simulink model "Simulate_v2"  (R2024b)
settings: Solver=VariableStepAuto  StartTime=0.0  StopTime=Tf  FixedStep=Ti  MaxStep=Ti  RelTol=1e-6
undefined symbols (not defined in the file): CCMPC, CEMPC, DiscIntNeverNeededParam, dspblkCoreblockFVToolHelper, FOC, gcbh, IM, LPF, M2C, plecs, PLL, RFT, TEB, Ti, Ts
libraries: slpidlib x4, dspstat3 x1, embmathops x1, spsabctodq0Lib x1, spsdq0toabcLib x1
settings Model: Creator=Pablo  LastModifiedBy=Pablo

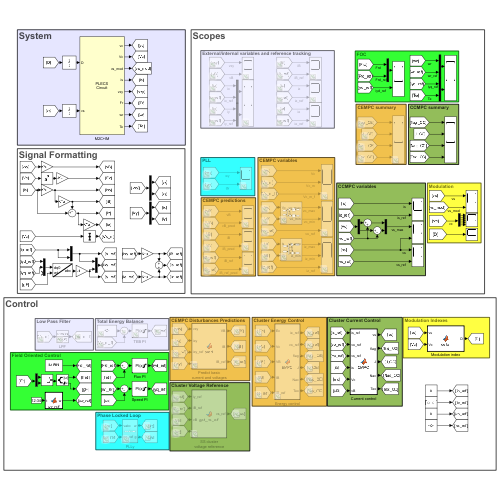
[thumbnail: Simulink's stored preview of the top-level diagram]
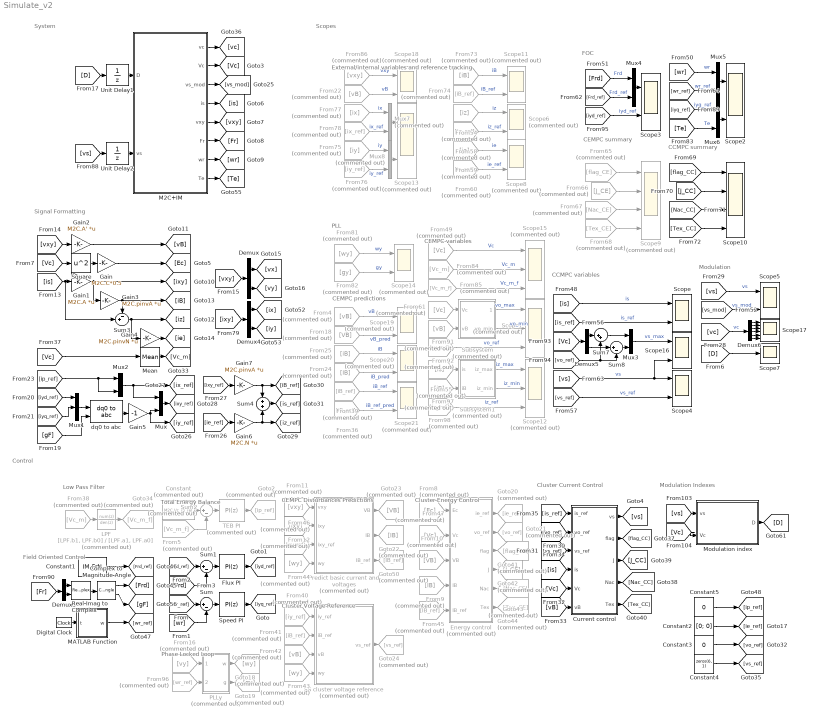
== system Simulate_v2 ==
  note: System
  note: Control
  note: Scopes
  note: External/internal variables and reference tracking
  note: CCMPC variables
  note: PLL
  note: CEMPC variables
  note: CEMPC predictions
  note: Modulation
  note: FOC
  note: CEMPC summary
  note: Cluster Current Control
  note: Cluster Voltage Reference
  note: Cluster Energy Control
  note: Signal Formatting
  note: CEMPC Disturbances Predictions
  note: Field Oriented Control
  note: Total Energy Balance
  note: Low Pass Filter
  note: Phase Locked Loop
  note: CCMPC summary
  note: Modulation Indexes
  Complex to Magnitude-Angle : ComplexToMagnitudeAngle
  Constant : Constant  Commented=on  Value=M2C.Vc_m_ref  SampleTime=Ts
  Constant1 : Constant  Value=IM.FrN  SampleTime=Ts
  Constant2 : Constant  Value=[0; 0]  SampleTime=Ts
  Constant3 : Constant  Value=0  SampleTime=Ts
  Constant4 : Constant  Value=zeros(6, 1)  SampleTime=Ts
  Constant5 : Constant  Value=0  SampleTime=Ts
  Current control : MATLAB Function  TreatAsAtomicUnit=on  SystemSampleTime=CCMPC.Ts
  Demux : Demux  Outputs=[2; 3]
  Demux3 : Demux  Outputs=2
  Demux4 : Demux  Outputs=[2; 3]
  Demux5 : Demux  Outputs=[3; 3]
  Demux6 : Demux  Outputs=M2C.m
  Digital Clock : DigitalClock  SampleTime=Ts
  Energy control : MATLAB Function  Commented=on  TreatAsAtomicUnit=on  SystemSampleTime=CEMPC.Ts
  Flux PI : slpidlib/PID Controller  Controller=PI  Form=Parallel  TimeDomain=Discrete-time  UseExternalTs=off  SampleTime=FOC.Ts  IntegratorMethod=Forward Euler  FilterMethod=Forward Euler  ControllerParametersSource=internal  P=FOC.kp_F  I=FOC.ki_F  UseKiTs=off  D=0  UseExternalDerivativeSource=off  N=100  UseFilter=on  TunerSelectOption=Transfer Function Based (PID Tuner App)  InitialConditionSource=internal  InitialConditionForIntegrator=0  InitialConditionForFilter=0  DifferentiatorICPrevScaledInput=0  ExternalReset=none  TrackingMode=off  Kt=1  LimitOutput=on  SatLimitsSource=internal  UpperSaturationLimit=FOC.u_max  LowerSaturationLimit=FOC.u_min  LinearizeAsGain=on  AntiWindupMode=back-calculation  Kb=FOC.kp_F  LimitIntegrator=off  UpperIntegratorSaturationLimit=inf  LowerIntegratorSaturationLimit=-inf  POutMin=[]  POutMax=[]  IOutMin=[]  IOutMax=[]  DOutMin=[]  DOutMax=[]  NOutMin=[]  NOutMax=[]  SumOutMin=[]  SumOutMax=[]  SaturationOutMin=[]  SaturationOutMax=[]  PParamMin=[]  PParamMax=[]  IParamMin=[]  IParamMax=[]  DParamMin=[]  DParamMax=[]  NParamMin=[]  NParamMax=[]  KbParamMin=[]  KbParamMax=[]  KtParamMin=[]  KtParamMax=[]  KbOutMin=[]  KbOutMax=[]  KtOutMin=[]  KtOutMax=[]  IntegratorOutMin=[]  IntegratorOutMax=[]  FilterOutMin=[]  FilterOutMax=[]  SumI1OutMin=[]  SumI1OutMax=[]  SumI2OutMin=[]  SumI2OutMax=[]  SumI3OutMin=[]  SumI3OutMax=[]  SumI4OutMin=[]  SumI4OutMax=[]  SumDOutMin=[]  SumDOutMax=[]  DifferentiatorOutMin=[]  DifferentiatorOutMax=[]  FilterDiffOutCoefMin=[]  FilterDiffOutCoefMax=[]  ReciprocalOutMin=[]  ReciprocalOutMax=[]  SumDenOutMin=[]  SumDenOutMax=[]  SumNumOutMin=[]  SumNumOutMax=[]  DivideOutMin=[]  DivideOutMax=[]  UdiffTsProdOutMin=[]  UdiffTsProdOutMax=[]  NTsProdOutMin=[]  NTsProdOutMax=[]  UintegralTsProdOutMin=[]  UintegralTsProdOutMax=[]  UngainTsProdOutMin=[]  UngainTsProdOutMax=[]  ClampingZeroOutDataTypeStr=Inherit: Inherit via back propagation  ClampingZeroOutMin=[]  ClampingZeroOutMax=[]  FilterDenConstantOutDataTypeStr=Inherit: Inherit via back propagation  FilterDenConstantOutMin=[]  FilterDenConstantOutMax=[]  PCopyOutDataTypeStr=Inherit: Inherit via back propagation  PCopyOutMin=[]  PCopyOutMax=[]  NCopyOutDataTypeStr=Inherit: Inherit via back propagation  NCopyOutMin=[]  NCopyOutMax=[]  IntegratorContinuousStateAttributes=''  IntegratorStateMustResolveToSignalObject=off  IntegratorRTWStateStorageClass=Auto  FilterContinuousStateAttributes=''  FilterStateMustResolveToSignalObject=off  FilterRTWStateStorageClass=Auto  ParallelPVariant=InternalParameters  IdealPVariant=Disabled  IVariant=InternalParameters  DVariant=Disabled  IntegratorVariant=Discrete  SatVariant=Enabled  AWVariant=BackCalculation  PCopyVariant=Disabled  TRVariant=Disabled  FdbkBlocksVariant=Forward  IdealPFdbkVariant=Disabled  SatFdbkVariant=Disabled  DerivativeFilterVariant=Disabled  NVariant=Disabled  NCopyVariant=Disabled_SignalSpec  FilterICVariant=Disabled  IntegratorICVariant=InternalICs  ExternalResetVariant=Disabled  TRSumVariant=Passthrough  SumFdbkVariant=Disabled  SumVariant=Sum_PI  TsampFilterVariant=InternalTs  TsampNgainVariant=Passthrough  TsampIntegralVariant=Disabled_SignalSpec  ExternalSaturationOutDataTypeStr=Inherit: Same as second input  DerivativeSourceVariant=Disabled  PreIntVariant=InternalPreInt
  From10 : From  Commented=on  GotoTag=VB
  From11 : From  Commented=on  GotoTag=vxy
  From12 : From  Commented=on  GotoTag=ixy
  From16 : From  Commented=on  GotoTag=vy
  From18 : From  Commented=on  GotoTag=VB
  From{4,22,42,91} (4 alike) : From  Commented=on  GotoTag=vB
  From24 : From  Commented=on  GotoTag=IB
  From25 : From  Commented=on  GotoTag=iB
  From36 : From  Commented=on  GotoTag=IB_ref
  From38 : From  Commented=on  GotoTag=Vc_m
  From39 : From  Commented=on  GotoTag=iB_ref
  From40 : From  Commented=on  GotoTag=iy_ref
  From41 : From  Commented=on  GotoTag=iB_ref
  From43 : From  Commented=on  GotoTag=wy
  From44 : From  Commented=on  GotoTag=wy
  From45 : From  Commented=on  GotoTag=IB_ref
  From46 : From  Commented=on  GotoTag=ixy_ref
  From47 : From  Commented=on  GotoTag=Vc
  From49 : From  Commented=on  GotoTag=Vc
  From5 : From  Commented=on  GotoTag=Vc_m_f
  From54 : From  Commented=on  GotoTag=iz
  From55 : From  Commented=on  GotoTag=is
  From58 : From  Commented=on  GotoTag=iz_ref
  From59 : From  Commented=on  GotoTag=ie
  From60 : From  Commented=on  GotoTag=ie_ref
  From61 : From  Commented=on  GotoTag=Vc
  From65 : From  Commented=on  GotoTag=flag_CE
  From66 : From  Commented=on  GotoTag=J_CE
  From67 : From  Commented=on  GotoTag=Nac_CE
  From68 : From  Commented=on  GotoTag=Tex_CE
  From73 : From  Commented=on  GotoTag=iB
  From74 : From  Commented=on  GotoTag=iB_ref
  From75 : From  Commented=on  GotoTag=iy
  From76 : From  Commented=on  GotoTag=iy_ref
  From77 : From  Commented=on  GotoTag=ix
  From78 : From  Commented=on  GotoTag=ix_ref
  From8 : From  Commented=on  GotoTag=Ec
  From81 : From  Commented=on  GotoTag=wy
  From82 : From  Commented=on  GotoTag=gy
  From84 : From  Commented=on  GotoTag=Vc_m
  From85 : From  Commented=on  GotoTag=Vc_m_f
  From86 : From  Commented=on  GotoTag=vxy
  From9 : From  Commented=on  GotoTag=IB
  From92 : From  Commented=on  GotoTag=vo_ref
  From96 : From  Commented=on  GotoTag=wr_ref
  From97 : From  Commented=on  GotoTag=iB
  From98 : From  Commented=on  GotoTag=iz_ref
  Gain : Gain  Gain=M2C.C*0.5
  Gain1 : Gain  Gain=M2C.A  Multiplication=Matrix(K*u)
  Gain2 : Gain  Gain=M2C.A'  Multiplication=Matrix(K*u)
  Gain3 : Gain  Gain=M2C.pinvA  Multiplication=Matrix(K*u)
  Gain4 : Gain  Gain=M2C.pinvN  Multiplication=Matrix(K*u)
  Gain5 : Gain  Gain=-1
  Gain6 : Gain  Gain=M2C.N  Multiplication=Matrix(K*u)
  Gain7 : Gain  Gain=M2C.pinvA  Multiplication=Matrix(K*u)
  Goto18 : Goto  Commented=on  GotoTag=wy
  Goto19 : Goto  Commented=on  GotoTag=gy
  Goto2 : Goto  Commented=on  GotoTag=ip_ref
  Goto20 : Goto  Commented=on  GotoTag=ie_ref
  Goto21 : Goto  Commented=on  GotoTag=vo_ref
  Goto22 : Goto  Commented=on  GotoTag=IB
  Goto23 : Goto  Commented=on  GotoTag=VB
  Goto24 : Goto  Commented=on  GotoTag=vs_ref
  Goto34 : Goto  Commented=on  GotoTag=Vc_m_f
  Goto41 : Goto  Commented=on  GotoTag=flag_CE
  Goto42 : Goto  Commented=on  GotoTag=J_CE
  Goto43 : Goto  Commented=on  GotoTag=Nac_CE
  Goto44 : Goto  Commented=on  GotoTag=Tex_CE
  Goto50 : Goto  Commented=on  GotoTag=IB_ref
  LPF : DiscreteTransferFcn  Commented=on  LoadFcn=dspblkCoreblockFVToolHelper(gcbh,'load');  Numerator=[LPF.b1, LPF.b0]  Denominator=[LPF.a1, LPF.a0]  InitialStates=M2C.Vc_m_ref*9.3230807
      settings: CopyFcn=dspblkCoreblockFVToolHelper(gcbh,'copy');  DeleteFcn=dspblkCoreblockFVToolHelper(gcbh,'close');  ModelCloseFcn=dspblkCoreblockFVToolHelper(gcbh,'close');  PreSaveFcn=dspblkCoreblockFVToolHelper(gcbh,'presave');  PostSaveFcn=dspblkCoreblockFVToolHelper(gcbh,'postsave');  CloseFcn=dspblkCoreblockFVToolHelper(gcbh,'close');
  M2C+IM : Subsystem  LoadFcn=plecs('sl', 200);  InitFcn=plecs('sl', 214);  StartFcn=plecs('sl', 208);  StopFcn=plecs('sl', 209);  mask(PlecsCircuit){PLECSData=<binary blob, 39888 chars, not shown>}
      mask prompts: PLECSData "PLECS Data (Do not delete or modify!)"
      mask init:
      | % PLACE CUSTOM INITIALIZATIONS ABOVE
      | % DO NOT REMOVE
      | plecs('sl', 215);
      | % DO NOT REMOVE
      settings: CopyFcn=plecs('sl', 203);  DeleteFcn=plecs('sl', 205);  UndoDeleteFcn=plecs('sl', 206);  PreSaveFcn=plecs('sl', 211);  PostSaveFcn=plecs('sl', 201);  NameChangeFcn=plecs('sl', 210);  DestroyFcn=plecs('sl', 207);  PreCopyFcn=plecs('sl', 216);  OpenFcn=plecs('sl', 202);  ErrorFcn=plerrorfcn
      mask Help: eval('plecs(''help'', ''qthelp:///creatingacircuit.html'')')
      mask Display: disp('PLECS\nCircuit')
  MATLAB Function : MATLAB Function  TreatAsAtomicUnit=on  SystemSampleTime=Ts
  Mean : dspstat3/Mean  run=off  InputProcessing=Columns as channels (frame based)  reset_popup=None  directionMode=Entire input  dimension=1  roiEnable=off  roiType=Rectangles  roiPortion=Entire ROI  roiOutput=Individual statistics for each ROI  roiFlag=off  roundingMode=Floor  overflowMode=off  outputDataTypeStr=Inherit: Same as accumulator  outputMin=[]  outputMax=[]  outputLastDataTypeStr=Inherit: Same as accumulator
  Modulation index : MATLAB Function  TreatAsAtomicUnit=on  SystemSampleTime=Ts
  Mux : Mux  Inputs=[M2C.p; M2C.q]
  Mux1 : Mux  Inputs=3
  Mux{2,4..6} (4 alike) : Mux  Inputs=2
  Mux3 : Mux  Inputs=[3; 3]
  Mux7 : Mux  Commented=on  Inputs=[2; 2]
  Mux8 : Mux  Commented=on  Inputs=[3; 3]
  PLLy : Subsystem  Commented=on
  Predict basic current and voltages : MATLAB Function  Commented=on  TreatAsAtomicUnit=on
  Real-Imag to Complex : RealImagToComplex
  SS cluster voltage reference : MATLAB Function  Commented=on  TreatAsAtomicUnit=on  SystemSampleTime=CCMPC.Ts
  Scope{,2..5,16} (6 alike) : Scope  NumInputPorts=2
  Scope1 : Scope  Commented=on  NumInputPorts=3
  Scope10 : Scope  NumInputPorts=4
  Scope{6,8,11,13..14,18..21} (9 alike) : Scope  Commented=on  NumInputPorts=2
  Scope12 : Scope  Commented=on  NumInputPorts=3
  Scope15 : Scope  Commented=on  NumInputPorts=3
  Scope17 : Scope  NumInputPorts=6
  Scope7 : Scope
  Scope9 : Scope  Commented=on  NumInputPorts=4
  Speed PI : slpidlib/PID Controller  Controller=PI  Form=Parallel  TimeDomain=Discrete-time  UseExternalTs=off  SampleTime=FOC.Ts  IntegratorMethod=Forward Euler  FilterMethod=Forward Euler  ControllerParametersSource=internal  P=FOC.kp_w  I=FOC.ki_w  UseKiTs=off  D=0  UseExternalDerivativeSource=off  N=100  UseFilter=on  TunerSelectOption=Transfer Function Based (PID Tuner App)  InitialConditionSource=internal  InitialConditionForIntegrator=0  InitialConditionForFilter=0  DifferentiatorICPrevScaledInput=0  ExternalReset=none  TrackingMode=off  Kt=1  LimitOutput=on  SatLimitsSource=internal  UpperSaturationLimit=FOC.u_max  LowerSaturationLimit=FOC.u_min  LinearizeAsGain=on  AntiWindupMode=clamping  Kb=1  LimitIntegrator=off  UpperIntegratorSaturationLimit=inf  LowerIntegratorSaturationLimit=-inf  POutMin=[]  POutMax=[]  IOutMin=[]  IOutMax=[]  DOutMin=[]  DOutMax=[]  NOutMin=[]  NOutMax=[]  SumOutMin=[]  SumOutMax=[]  SaturationOutMin=[]  SaturationOutMax=[]  PParamMin=[]  PParamMax=[]  IParamMin=[]  IParamMax=[]  DParamMin=[]  DParamMax=[]  NParamMin=[]  NParamMax=[]  KbParamMin=[]  KbParamMax=[]  KtParamMin=[]  KtParamMax=[]  KbOutMin=[]  KbOutMax=[]  KtOutMin=[]  KtOutMax=[]  IntegratorOutMin=[]  IntegratorOutMax=[]  FilterOutMin=[]  FilterOutMax=[]  SumI1OutMin=[]  SumI1OutMax=[]  SumI2OutMin=[]  SumI2OutMax=[]  SumI3OutMin=[]  SumI3OutMax=[]  SumI4OutMin=[]  SumI4OutMax=[]  SumDOutMin=[]  SumDOutMax=[]  DifferentiatorOutMin=[]  DifferentiatorOutMax=[]  FilterDiffOutCoefMin=[]  FilterDiffOutCoefMax=[]  ReciprocalOutMin=[]  ReciprocalOutMax=[]  SumDenOutMin=[]  SumDenOutMax=[]  SumNumOutMin=[]  SumNumOutMax=[]  DivideOutMin=[]  DivideOutMax=[]  UdiffTsProdOutMin=[]  UdiffTsProdOutMax=[]  NTsProdOutMin=[]  NTsProdOutMax=[]  UintegralTsProdOutMin=[]  UintegralTsProdOutMax=[]  UngainTsProdOutMin=[]  UngainTsProdOutMax=[]  ClampingZeroOutDataTypeStr=Inherit: Inherit via back propagation  ClampingZeroOutMin=[]  ClampingZeroOutMax=[]  FilterDenConstantOutDataTypeStr=Inherit: Inherit via back propagation  FilterDenConstantOutMin=[]  FilterDenConstantOutMax=[]  PCopyOutDataTypeStr=Inherit: Inherit via back propagation  PCopyOutMin=[]  PCopyOutMax=[]  NCopyOutDataTypeStr=Inherit: Inherit via back propagation  NCopyOutMin=[]  NCopyOutMax=[]  IntegratorContinuousStateAttributes=''  IntegratorStateMustResolveToSignalObject=off  IntegratorRTWStateStorageClass=Auto  FilterContinuousStateAttributes=''  FilterStateMustResolveToSignalObject=off  FilterRTWStateStorageClass=Auto  ParallelPVariant=InternalParameters  IdealPVariant=Disabled  IVariant=InternalParameters  DVariant=Disabled  IntegratorVariant=Discrete  SatVariant=Enabled  AWVariant=DiscClampingParallel  PCopyVariant=Disabled  TRVariant=Disabled  FdbkBlocksVariant=Forward  IdealPFdbkVariant=Disabled  SatFdbkVariant=Disabled  DerivativeFilterVariant=Disabled  NVariant=Disabled  NCopyVariant=Disabled_SignalSpec  FilterICVariant=Disabled  IntegratorICVariant=InternalICs  ExternalResetVariant=Disabled  TRSumVariant=Passthrough  SumFdbkVariant=Disabled  SumVariant=Sum_PI  TsampFilterVariant=InternalTs  TsampNgainVariant=Passthrough  TsampIntegralVariant=Disabled_SignalSpec  ExternalSaturationOutDataTypeStr=Inherit: Same as second input  DerivativeSourceVariant=Disabled  PreIntVariant=InternalPreInt
  Square : Math  Operator=square
  Subsystem : Subsystem  Commented=on
  Subsystem1 : Subsystem  Commented=on
  Sum : Sum  Inputs=|+-
  Sum1 : Sum  Inputs=|+-
  Sum2 : Sum  Commented=on  Inputs=|+-
  Sum3 : Sum  Inputs=-+|
  Sum4 : Sum
  Sum7 : Sum  Inputs=|++
  Sum8 : Sum  Inputs=|+-
  TEB PI : slpidlib/PID Controller  Commented=on  Controller=PI  Form=Parallel  TimeDomain=Discrete-time  UseExternalTs=off  SampleTime=TEB.Ts  IntegratorMethod=Forward Euler  FilterMethod=Forward Euler  ControllerParametersSource=internal  P=TEB.kp  I=TEB.ki  UseKiTs=off  D=0  UseExternalDerivativeSource=off  N=100  UseFilter=on  TunerSelectOption=Transfer Function Based (PID Tuner App)  InitialConditionSource=internal  InitialConditionForIntegrator=0  InitialConditionForFilter=0  DifferentiatorICPrevScaledInput=0  ExternalReset=none  TrackingMode=off  Kt=1  LimitOutput=on  SatLimitsSource=internal  UpperSaturationLimit=TEB.u_max  LowerSaturationLimit=TEB.u_min  LinearizeAsGain=on  AntiWindupMode=clamping  Kb=1  LimitIntegrator=off  UpperIntegratorSaturationLimit=inf  LowerIntegratorSaturationLimit=-inf  POutMin=[]  POutMax=[]  IOutMin=[]  IOutMax=[]  DOutMin=[]  DOutMax=[]  NOutMin=[]  NOutMax=[]  SumOutMin=[]  SumOutMax=[]  SaturationOutMin=[]  SaturationOutMax=[]  PParamMin=[]  PParamMax=[]  IParamMin=[]  IParamMax=[]  DParamMin=[]  DParamMax=[]  NParamMin=[]  NParamMax=[]  KbParamMin=[]  KbParamMax=[]  KtParamMin=[]  KtParamMax=[]  KbOutMin=[]  KbOutMax=[]  KtOutMin=[]  KtOutMax=[]  IntegratorOutMin=[]  IntegratorOutMax=[]  FilterOutMin=[]  FilterOutMax=[]  SumI1OutMin=[]  SumI1OutMax=[]  SumI2OutMin=[]  SumI2OutMax=[]  SumI3OutMin=[]  SumI3OutMax=[]  SumI4OutMin=[]  SumI4OutMax=[]  SumDOutMin=[]  SumDOutMax=[]  DifferentiatorOutMin=[]  DifferentiatorOutMax=[]  FilterDiffOutCoefMin=[]  FilterDiffOutCoefMax=[]  ReciprocalOutMin=[]  ReciprocalOutMax=[]  SumDenOutMin=[]  SumDenOutMax=[]  SumNumOutMin=[]  SumNumOutMax=[]  DivideOutMin=[]  DivideOutMax=[]  UdiffTsProdOutMin=[]  UdiffTsProdOutMax=[]  NTsProdOutMin=[]  NTsProdOutMax=[]  UintegralTsProdOutMin=[]  UintegralTsProdOutMax=[]  UngainTsProdOutMin=[]  UngainTsProdOutMax=[]  ClampingZeroOutDataTypeStr=Inherit: Inherit via back propagation  ClampingZeroOutMin=[]  ClampingZeroOutMax=[]  FilterDenConstantOutDataTypeStr=Inherit: Inherit via back propagation  FilterDenConstantOutMin=[]  FilterDenConstantOutMax=[]  PCopyOutDataTypeStr=Inherit: Inherit via back propagation  PCopyOutMin=[]  PCopyOutMax=[]  NCopyOutDataTypeStr=Inherit: Inherit via back propagation  NCopyOutMin=[]  NCopyOutMax=[]  IntegratorContinuousStateAttributes=''  IntegratorStateMustResolveToSignalObject=off  IntegratorRTWStateStorageClass=Auto  FilterContinuousStateAttributes=''  FilterStateMustResolveToSignalObject=off  FilterRTWStateStorageClass=Auto  ParallelPVariant=InternalParameters  IdealPVariant=Disabled  IVariant=InternalParameters  DVariant=Disabled  IntegratorVariant=Discrete  SatVariant=Enabled  AWVariant=DiscClampingParallel  PCopyVariant=Disabled  TRVariant=Disabled  FdbkBlocksVariant=Forward  IdealPFdbkVariant=Disabled  SatFdbkVariant=Disabled  DerivativeFilterVariant=Disabled  NVariant=Disabled  NCopyVariant=Disabled_SignalSpec  FilterICVariant=Disabled  IntegratorICVariant=InternalICs  ExternalResetVariant=Disabled  TRSumVariant=Passthrough  SumFdbkVariant=Disabled  SumVariant=Sum_PI  TsampFilterVariant=InternalTs  TsampNgainVariant=Passthrough  TsampIntegralVariant=Disabled_SignalSpec  ExternalSaturationOutDataTypeStr=Inherit: Same as second input  DerivativeSourceVariant=Disabled  PreIntVariant=InternalPreInt
  Unit Delay1 : UnitDelay  InitialCondition=zeros(6, 1)  SampleTime=Ti  HasFrameUpgradeWarning=on
  Unit Delay2 : UnitDelay  InitialCondition=zeros(6, 1)  SampleTime=Ti  HasFrameUpgradeWarning=on
  dq0 to abc : spsdq0toabcLib/dq0 to abc  Alignment=Aligned with phase A axis
  wires:
  [wr_ref] -> Sum/1
  [wr] -> Sum/2
  [Frd] -> Sum1/2
  [Frd_ref] -> Sum1/1
  Constant/1 -> Sum2/1
  Sum2/1 -> TEB PI/1
  TEB PI/1 -> Goto2/1
  M2C+IM/2(Vc) -> [Vc]
  Current control/1(vs) -> [vs]
  M2C+IM/3(vs_mod) -> [vs_mod]
  M2C+IM/5(vxy) -> [vxy]
  M2C+IM/6(Fr) -> [Fr]
  M2C+IM/7(wr) -> [wr]
  From8/1 -> Energy control/1(Ec)
  From9/1 -> Energy control/4(IB)
  From10/1 -> Energy control/3(VB)
  From12/1 -> Predict basic current and voltages/2(ixy)
  From11/1 -> Predict basic current and voltages/1(vxy)
  From16/1 -> PLLy/1(vabc)
  PLLy/1(w) -> Goto18/1
  PLLy/2(g) -> Goto19/1
  Energy control/1(ie_ref) -> Goto20/1
  SS cluster voltage reference/1(vs_ref) -> Goto24/1
  [vo_ref] -> Current control/2(vo_ref)
  [vs_ref] -> Current control/3(vs_ref)
  [Vc] -> Current control/5(Vc)
  [vB] -> Current control/6(vB)
  [is] -> Current control/4(is)
  [is_ref] -> Current control/1(is_ref)
  From5/1 -> Sum2/2
  From40/1 -> SS cluster voltage reference/1(iy_ref)
  From42/1 -> SS cluster voltage reference/3(vB)
  From41/1 -> SS cluster voltage reference/2(iB_ref)
  From43/1 -> SS cluster voltage reference/4(wy)
  M2C+IM/1(vc) -> [vc]
  From44/1 -> Predict basic current and voltages/4(wy)
  Current control/2(flag) -> [flag_CC]
  Current control/3(J) -> [J_CC]
  Current control/4(Nac) -> [Nac_CC]
  Current control/5(Tex) -> [Tex_CC]
  From45/1 -> Energy control/5(IB_ref)
  Energy control/2(vo_ref) -> Goto21/1
  From46/1 -> Predict basic current and voltages/3(ixy_ref)
  Predict basic current and voltages/3(IB_ref) -> Goto50/1
  Mux/1 -> [ixy_ref]
  [vxy] -> Demux/1
  Square/1 -> Gain/1
  [vxy] -> Gain2/1
  Gain1/1 -> [ixy], Gain3/1
  Mean/1 -> [Vc_m]
  Sum3/1 -> Gain4/1, [iz]
  Mux2/1 -> Mux/1, [ix_ref]
  Demux/2 -> [vy]
  Gain2/1 -> [vB]
  [ixy_ref] -> Gain7/1
  [is] -> Sum3/2, Gain1/1
  [Vc] -> Mean/1
  Demux/1 -> [vx]
  [ie_ref] -> Gain6/1
  [gF] -> dq0 to abc/2
  Gain3/1 -> [iB], Sum3/1
  dq0 to abc/1 -> Gain5/1
  Gain/1 -> [Ec]
  Sum4/1 -> [is_ref]
  [Vc] -> Square/1
  Gain4/1 -> [ie]
  Mux1/1 -> dq0 to abc/1
  From47/1 -> Energy control/2(Vc)
  From49/1 -> Scope15/1  "Vc"
  [vs_mod] -> Scope5/2  "vs_mod"
  Energy control/5(Nac) -> Goto43/1
  Energy control/6(Tex) -> Goto44/1
  Energy control/3(flag) -> Goto41/1
  Energy control/4(J) -> Goto42/1
  Predict basic current and voltages/1(VB) -> Goto23/1
  Predict basic current and voltages/2(IB) -> Goto22/1
  [vs_ref] -> Scope4/2  "vs_ref"
  From58/1 -> Scope6/2  "iz_ref"
  From54/1 -> Scope6/1  "iz"
  From59/1 -> Scope8/1  "ie"
  From60/1 -> Scope8/2  "ie_ref"
  Constant1/1 -> [Frd_ref]
  MATLAB Function/1(w) -> [wr_ref]
  From65/1 -> Scope9/1
  From66/1 -> Scope9/2
  From67/1 -> Scope9/3
  From68/1 -> Scope9/4
  [Tex_CC] -> Scope10/4
  [Nac_CC] -> Scope10/3
  [J_CC] -> Scope10/2
  [flag_CC] -> Scope10/1
  From74/1 -> Scope11/2  "iB_ref"
  From73/1 -> Scope11/1  "iB"
  [ixy] -> Demux4/1
  Demux4/1 -> [ix]
  Demux4/2 -> [iy]
  From82/1 -> Scope14/2  "gy"
  From81/1 -> Scope14/1  "wy"
  M2C+IM/8(Te) -> [Te]
  From84/1 -> Scope15/2  "Vc_m"
  From85/1 -> Scope15/3  "Vc_m_f"
  From86/1 -> Scope18/1  "vxy"
  Complex to Magnitude-Angle/1 -> [Frd]
  [iyq_ref] -> Mux1/2
  Gain7/1 -> Sum4/1, [iB_ref]
  Gain6/1 -> [iz_ref], Sum4/2
  From22/1 -> Scope18/2  "vB"
  M2C+IM/4(is) -> [is]
  [vs] -> Scope5/1  "vs"
  [vs] -> Scope16/2, Scope4/1  "vs"
  Complex to Magnitude-Angle/2 -> [gF]
  Demux3/2 -> Real-Imag to Complex/2
  Demux3/1 -> Real-Imag to Complex/1
  [Fr] -> Demux3/1
  Real-Imag to Complex/1 -> Complex to Magnitude-Angle/1
  Unit Delay1/1 -> M2C+IM/1(D)
  From38/1 -> LPF/1
  From4/1 -> Scope19/1  "vB"
  From18/1 -> Scope19/2  "vB_pred"
  From24/1 -> Scope20/2  "iB_pred"
  From25/1 -> Scope20/1  "iB"
  From36/1 -> Scope21/2  "iB_ref_pred"
  From39/1 -> Scope21/1  "iB_ref"
  Gain5/1 -> [iy_ref], Mux/2
  From92/1 -> Scope1/3  "vo_ref"
  [Vc] -> Demux5/1
  Demux5/1 -> Sum7/1
  Demux5/2 -> Sum8/1
  [vo_ref] -> Sum7/2, Sum8/2
  Sum7/1 -> Mux3/1
  Sum8/1 -> Mux3/2
  Mux3/1 -> Scope16/1  "vs_max"
  [ip_ref] -> Mux2/2, Mux2/1
  LPF/1 -> Goto34/1
  [iyd_ref] -> Mux1/1
  [vc] -> Demux6/1  "vc"
  Digital Clock/1 -> MATLAB Function/1(t)
  Sum1/1 -> Flux PI/1
  Sum/1 -> Speed PI/1
  Flux PI/1 -> [iyd_ref]
  Speed PI/1 -> [iyq_ref]
  Constant2/1 -> [ie_ref]
  Constant3/1 -> [vo_ref]
  Constant4/1 -> [vs_ref]
  [iyd_ref] -> Scope3/2  "iyd_ref"
  From96/1 -> PLLy/2(wr_ref)
  [Frd] -> Mux4/1  "Frd"
  [Frd_ref] -> Mux4/2  "Frd_ref"
  Mux4/1 -> Scope3/1
  [wr] -> Mux5/1  "wr"
  [wr_ref] -> Mux5/2  "wr_ref"
  Mux5/1 -> Scope2/1
  [Te] -> Mux6/2  "Te"
  [iyq_ref] -> Mux6/1  "iyq_ref"
  Mux6/1 -> Scope2/2
  [D] -> Unit Delay1/1
  From77/1 -> Mux7/1  "ix"
  From78/1 -> Mux7/2  "ix_ref"
  From75/1 -> Mux8/1  "iy"
  From76/1 -> Mux8/2  "iy_ref"
  Mux7/1 -> Scope13/1
  Mux8/1 -> Scope13/2
  From61/1 -> Subsystem/1(Vc)
  From91/1 -> Subsystem/2(vB)
  Subsystem/1(vo_max) -> Scope1/1  "vo_max"
  Subsystem/2(vo_min) -> Scope1/2  "vo_min"
  Subsystem1/2(iz_min) -> Scope12/2  "iz_min"
  Subsystem1/1(iz_max) -> Scope12/1  "iz_max"
  From97/1 -> Subsystem1/2(iB)
  From55/1 -> Subsystem1/1(is)
  From98/1 -> Scope12/3  "iz_ref"
  Constant5/1 -> [ip_ref]
  [is] -> Scope/1  "is"
  [is_ref] -> Scope/2  "is_ref"
  Modulation index/1(D) -> [D]
  [vs] -> Modulation index/1(vs)
  [Vc] -> Modulation index/2(Vc)
  [vs] -> Unit Delay2/1
  Unit Delay2/1 -> M2C+IM/2(vs)
  [D] -> Scope7/1
  Demux6/1 -> Scope17/1
  Demux6/2 -> Scope17/2
  Demux6/3 -> Scope17/3
  Demux6/4 -> Scope17/4
  Demux6/5 -> Scope17/5
  Demux6/6 -> Scope17/6

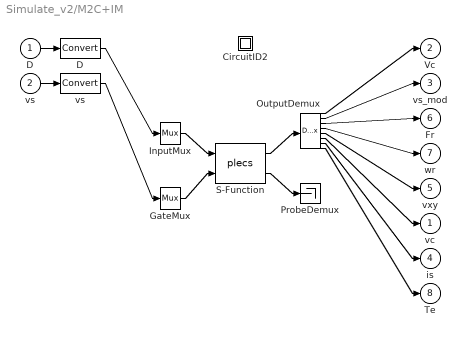
== system Simulate_v2/M2C+IM ==
  D : Inport  PortDimensions=6
  vs : Inport  Port=2  PortDimensions=6
  " CircuitID2 " : Subsystem
  " D " : DataTypeConversion
  " GateMux " : Mux  Inputs=[ 6 ]
  " InputMux " : Mux  Inputs=[ 6 ]
  " OutputDemux " : Demux  Outputs=[ 6 6 2 1 5 24 6 1 ]
  " ProbeDemux " : Terminator
  " S-Function " : S-Function  FunctionName=plecs  SFunctionDeploymentMode=off  EnableBusSupport=off
  " vs " : DataTypeConversion
  vc : Outport  PortDimensions=24
  Vc : Outport  Port=2  PortDimensions=6
  vs_mod : Outport  Port=3  PortDimensions=6
  is : Outport  Port=4  PortDimensions=6
  vxy : Outport  Port=5  PortDimensions=5
  Fr : Outport  Port=6  PortDimensions=2
  wr : Outport  Port=7  PortDimensions=1
  Te : Outport  Port=8  PortDimensions=1
  wires:
  " InputMux "/1 -> " S-Function "/1
  " GateMux "/1 -> " S-Function "/2
  " S-Function "/1 -> " OutputDemux "/1
  " S-Function "/2 -> " ProbeDemux "/1
  D/1 -> " D "/1
  " D "/1 -> " InputMux "/1
  vs/1 -> " vs "/1
  " vs "/1 -> " GateMux "/1
  " OutputDemux "/1 -> Vc/1
  " OutputDemux "/2 -> vs_mod/1
  " OutputDemux "/3 -> Fr/1
  " OutputDemux "/4 -> wr/1
  " OutputDemux "/5 -> vxy/1
  " OutputDemux "/6 -> vc/1
  " OutputDemux "/7 -> is/1
  " OutputDemux "/8 -> Te/1

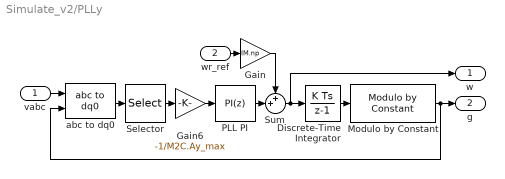
== system Simulate_v2/PLLy ==
  vabc : Inport
  wr_ref : Inport  Port=2
  Discrete-Time Integrator : DiscreteIntegrator  SampleTime=PLL.Ts  ICPrevOutput=DiscIntNeverNeededParam  ICPrevScaledInput=DiscIntNeverNeededParam
  Gain : Gain  Gain=IM.np
  Gain6 : Gain  Gain=-1/M2C.Ay_max
  Modulo by Constant : embmathops/Modulo by Constant  Denominator=2*pi  SimulateUsing=Code generation
      settings: LibrarySourceBlock=embeddedMathLib/Modulo by Constant
  PLL PI : slpidlib/PID Controller  Controller=PI  Form=Parallel  TimeDomain=Discrete-time  UseExternalTs=off  SampleTime=PLL.Ts  IntegratorMethod=Forward Euler  FilterMethod=Forward Euler  ControllerParametersSource=internal  P=PLL.kp  I=PLL.ki  UseKiTs=off  D=0  UseExternalDerivativeSource=off  N=100  UseFilter=on  TunerSelectOption=Transfer Function Based (PID Tuner App)  InitialConditionSource=internal  InitialConditionForIntegrator=0  InitialConditionForFilter=0  DifferentiatorICPrevScaledInput=0  ExternalReset=none  TrackingMode=off  Kt=1  LimitOutput=off  SatLimitsSource=internal  UpperSaturationLimit=inf  LowerSaturationLimit=-inf  LinearizeAsGain=on  AntiWindupMode=none  Kb=1  LimitIntegrator=off  UpperIntegratorSaturationLimit=inf  LowerIntegratorSaturationLimit=-inf  POutMin=[]  POutMax=[]  IOutMin=[]  IOutMax=[]  DOutMin=[]  DOutMax=[]  NOutMin=[]  NOutMax=[]  SumOutMin=[]  SumOutMax=[]  SaturationOutMin=[]  SaturationOutMax=[]  PParamMin=[]  PParamMax=[]  IParamMin=[]  IParamMax=[]  DParamMin=[]  DParamMax=[]  NParamMin=[]  NParamMax=[]  KbParamMin=[]  KbParamMax=[]  KtParamMin=[]  KtParamMax=[]  KbOutMin=[]  KbOutMax=[]  KtOutMin=[]  KtOutMax=[]  IntegratorOutMin=[]  IntegratorOutMax=[]  FilterOutMin=[]  FilterOutMax=[]  SumI1OutMin=[]  SumI1OutMax=[]  SumI2OutMin=[]  SumI2OutMax=[]  SumI3OutMin=[]  SumI3OutMax=[]  SumI4OutMin=[]  SumI4OutMax=[]  SumDOutMin=[]  SumDOutMax=[]  DifferentiatorOutMin=[]  DifferentiatorOutMax=[]  FilterDiffOutCoefMin=[]  FilterDiffOutCoefMax=[]  ReciprocalOutMin=[]  ReciprocalOutMax=[]  SumDenOutMin=[]  SumDenOutMax=[]  SumNumOutMin=[]  SumNumOutMax=[]  DivideOutMin=[]  DivideOutMax=[]  UdiffTsProdOutMin=[]  UdiffTsProdOutMax=[]  NTsProdOutMin=[]  NTsProdOutMax=[]  UintegralTsProdOutMin=[]  UintegralTsProdOutMax=[]  UngainTsProdOutMin=[]  UngainTsProdOutMax=[]  ClampingZeroOutDataTypeStr=Inherit: Inherit via back propagation  ClampingZeroOutMin=[]  ClampingZeroOutMax=[]  FilterDenConstantOutDataTypeStr=Inherit: Inherit via back propagation  FilterDenConstantOutMin=[]  FilterDenConstantOutMax=[]  PCopyOutDataTypeStr=Inherit: Inherit via back propagation  PCopyOutMin=[]  PCopyOutMax=[]  NCopyOutDataTypeStr=Inherit: Inherit via back propagation  NCopyOutMin=[]  NCopyOutMax=[]  IntegratorContinuousStateAttributes=''  IntegratorStateMustResolveToSignalObject=off  IntegratorRTWStateStorageClass=Auto  FilterContinuousStateAttributes=''  FilterStateMustResolveToSignalObject=off  FilterRTWStateStorageClass=Auto  ParallelPVariant=InternalParameters  IdealPVariant=Disabled  IVariant=InternalParameters  DVariant=Disabled  IntegratorVariant=Discrete  SatVariant=Disabled  AWVariant=Passthrough  PCopyVariant=Disabled  TRVariant=Disabled  FdbkBlocksVariant=Forward  IdealPFdbkVariant=Disabled  SatFdbkVariant=Disabled  DerivativeFilterVariant=Disabled  NVariant=Disabled  NCopyVariant=Disabled_SignalSpec  FilterICVariant=Disabled  IntegratorICVariant=InternalICs  ExternalResetVariant=Disabled  TRSumVariant=Passthrough  SumFdbkVariant=Disabled  SumVariant=Sum_PI  TsampFilterVariant=InternalTs  TsampNgainVariant=Passthrough  TsampIntegralVariant=Disabled_SignalSpec  ExternalSaturationOutDataTypeStr=Inherit: Same as second input  DerivativeSourceVariant=Disabled  PreIntVariant=InternalPreInt
  Selector : Selector  InputPortWidth=3  IndexOptions=Index vector (dialog)  Indices=[2]  OutputSizes=1
  Sum : Sum  Inputs=++|
  abc to dq0 : spsabctodq0Lib/abc to dq0  Alignment=Aligned with phase A axis
  w : Outport
  g : Outport  Port=2
  wires:
  Gain6/1 -> PLL PI/1
  Discrete-Time Integrator/1 -> Modulo by Constant/1
  abc to dq0/1 -> Selector/1
  Selector/1 -> Gain6/1
  vabc/1 -> abc to dq0/1
  Modulo by Constant/1 -> abc to dq0/2, g/1
  PLL PI/1 -> Sum/2
  Sum/1 -> w/1, Discrete-Time Integrator/1
  wr_ref/1 -> Gain/1
  Gain/1 -> Sum/1

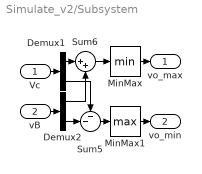
== system Simulate_v2/Subsystem ==
  Vc : Inport
  vB : Inport  Port=2
  Demux1 : Demux  Outputs=[3; 3]
  Demux2 : Demux  Outputs=[3; 3]
  MinMax : MinMax
  MinMax1 : MinMax  Function=max
  Sum5 : Sum  Inputs=--|
  Sum6 : Sum  Inputs=|++
  vo_max : Outport
  vo_min : Outport  Port=2
  wires:
  Sum5/1 -> MinMax1/1
  Sum6/1 -> MinMax/1
  Demux2/2 -> Sum5/2
  Demux1/2 -> Sum5/1
  Demux2/1 -> Sum6/2
  MinMax/1 -> vo_max/1
  Demux1/1 -> Sum6/1
  Vc/1 -> Demux1/1
  MinMax1/1 -> vo_min/1
  vB/1 -> Demux2/1

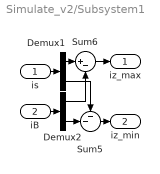
== system Simulate_v2/Subsystem1 ==
  is : Inport
  iB : Inport  Port=2
  Demux1 : Demux  Outputs=[3; 3]
  Demux2 : Demux  Outputs=[3; 3]
  Sum5 : Sum  Inputs=--|
  Sum6 : Sum  Inputs=|+-
  iz_max : Outport
  iz_min : Outport  Port=2
  wires:
  Demux2/2 -> Sum5/2
  Demux1/2 -> Sum5/1
  Demux2/1 -> Sum6/2
  Sum6/1 -> iz_max/1
  Demux1/1 -> Sum6/1
  is/1 -> Demux1/1
  Sum5/1 -> iz_min/1
  iB/1 -> Demux2/1

== system Simulate_v2/M2C+IM/ CircuitID2  ==

== matlab function Simulate_v2/Energy control ==
  data: Ec input; Vc input; VB input; IB input; IB_ref input; ie_ref output; vo_ref output; flag output; J output; Nac output; Tex output; M2C parameter; CEMPC parameter
function [ie_ref, vo_ref, flag, J, Nac, Tex] = EMPC(Ec, Vc, VB, IB, IB_ref, M2C, CEMPC)
%#codegen

Ec_m_ref = 0;
flag_i = int32(0);
flag_v = int32(0);

persistent Ts m n Np NN ONE_n Nl is_max Vc_m_ref Hu_i Aineq_i lambda_i Hu_v Aineq_v lambda_v iA_i iA_v options_i options_v
if isempty(iA_i)
Ts = CEMPC.Ts;
m = M2C.m;
n = M2C.n;
Np = CEMPC.Np;
NN = CEMPC.NN;
ONE_n = CEMPC.ONE_n;
Nl = CEMPC.Nl;
is_max = M2C.is_max;
Vc_m_ref = M2C.Vc_m_ref;
Ec_m_ref = M2C.Ec_m_ref;
Hu_i = CEMPC.Hu_i;
Aineq_i = CEMPC.Aineq_i;
lambda_i = CEMPC.lambda_i;
Hu_v = CEMPC.Hu_v;
Aineq_v = CEMPC.Aineq_v;
lambda_v = CEMPC.lambda_v;
iA_i = false(size(zeros(2 * m * Np, 1)));
iA_v = false(size(zeros(2 * Np, 1)));
options_i                     = mpcActiveSetOptions;
options_i.MaxIterations       = 20;
options_i.ConstraintTolerance = 1e-4;
options_v                     = mpcActiveSetOptions;
options_v.MaxIterations       = 10;
options_v.ConstraintTolerance = 1e-4;
end

tic

% Initialize common mode voltage vector of horizon Np
vo_ref_temp = zeros(Np, 1);
ie_ref_temp = zeros(n * Np, 1);
vs_temp = zeros(m * Np, 1);
is_temp = zeros(m * Np, 1);

for l = 1:Nl
    %%% Circulating currents subproblem Jz = Jz_x + Jz_u

    % Initialization
    vs_temp = VB(:) + ONE_n * vo_ref_temp;

    % Formulation

    % Control action penalization Jz_u
    fu_i = 2 * (NN') * IB(:);
    fu_i = fu_i / is_max^2;

    % Constraints
    ub      =  is_max - IB_ref(:);
    lb      = -is_max - IB_ref(:);
    bineq_i = [ub; -lb];

    % Solve
    [ie_ref_temp, flag_i, iA_i, ~] = solve_subproblem(Ec, vs_temp, IB(:), NN, Hu_i, fu_i, Aineq_i, bineq_i, lambda_i, iA_i, options_i, CEMPC, M2C);

    %%% Common mode voltage subproblem Jo = Jo_x + Jo_u

    % Initialization
    is_temp = IB(:) + NN * ie_ref_temp;

    % Formulation

    % Control action penalization Jo_u
    fu_v = zeros(Np, 1);
    fu_v = fu_v / Vc_m_ref^2;

    % Constraints
    ub = min(Vc(1:3) - VB(1:3, :), [], 1)';
    lb = max(-Vc(4:6) - VB(4:6, :), [], 1)';
    bineq_v = [ub; -lb];

    % Solve
    [vo_ref_temp, flag_v, iA_v, ~] = solve_subproblem(Ec, is_temp, VB(:), ONE_n, Hu_v, fu_v, Aineq_v, bineq_v, lambda_v, iA_v, options_v, CEMPC, M2C);
    vs_temp = VB(:) + ONE_n * vo_ref_temp;
end

% ie_ref = ie_ref_temp(1:n);
ie_ref = ie_ref_temp(1:2);
vo_ref = vo_ref_temp(1);

if and(0 < flag_i, 0 < flag_v)
    flag_T = 1;
else
    flag_T = -3;
end

Ec_pred = Ec + Ts * reshape(vs_temp .* is_temp, m, Np);
Ec_pred = Ec_pred(:);
J_E = sum((Ec_pred - mean(Ec_pred)).^2) / Ec_m_ref^2;
J_i = sum(is_temp.^2) / is_max^2;
J_v = sum(vo_ref_temp.^2) / Vc_m_ref^2;
J_T = J_E + lambda_i * J_i + lambda_v * J_v;

flag = [flag_i, flag_v, flag_T];
J = [J_E, J_i, J_v, J_T];
Nac = [sum(iA_i), sum(iA_v)];

Tex = toc;
end

function [Uopt, exitflag, iA, mu] = solve_subproblem(x, var_s, P, Maux, Hu, fu, Aineq, bineq, lambda, iA, options, CEMPC, M2C)
    % solve_subproblem: Find Uopt which brings state variables close to its mean

    % Suitable for any input affine system. (The model for each block
    % in BCD is input affine).
    % Model: X[t+1:t+Np-1] = A * x[t] + B * U[t:t+Np-1] + E * P[t:t+Np-1]

    % Cost function: J = ||X[t+1:t+Np-1] - mean(X)[t+1:t+Np-1]||^2
    %                J = ||(I-1*1'/m)*X[t+1:t+Np-1]||^2 = ||IM*X[t+1:t+Np-1]||^2
    %                J = X' * IM' * IM * X = X' * IM2 * X

    E = CEMPC.Ts * CEMPC.K * diag(var_s);
    B = E * Maux;
    % Hx = 2 * (B') * CEMPC.IM2 * B;
    % fx = 2 * (B') * CEMPC.IM2 * (repmat(x, CEMPC.Np, 1) + E * P);
    Hx = 2 * (B') * B;
    fx = 2 * (B') * (repmat(x-mean(x), CEMPC.Np, 1) + E * P);
    Hx = Hx / M2C.Ec_m_ref^2;
    fx = fx / M2C.Ec_m_ref^2;
    H = Hx + lambda * Hu;
    f = fx + lambda * fu;
    H = (H + H') / 2;
    [Uopt, exitflag, iA, mu] = mpcActiveSetSolver(H, f, Aineq, bineq, zeros(0, size(Maux, 2)), zeros(0, 1), iA, options);
end

== matlab function Simulate_v2/Current control ==
  data: is_ref input; vo_ref input; vs_ref input; is input; vs output; Vc input; vB input; flag output; J output; Nac output; Tex output; M2C parameter; CCMPC parameter
function [vs, flag, J, Nac, Tex] = CMPC(is_ref, vo_ref, vs_ref, is, Vc, vB, M2C, CCMPC)
%#codegen

% vs: control action
% flag: solver verbose
% J: cost function
% Nac: # of active constraints
% Tex: Execution time

persistent one_n Ad Bd is_max Vc_m_ref lambda m H Aineq iA options
if isempty(one_n)
    one_n = [ones(3, 1); -ones(3, 1)];
    Ad = CCMPC.Ad;
    Bd = CCMPC.Bd;
    is_max = M2C.is_max;
    Vc_m_ref = M2C.Vc_m_ref;
    lambda = CCMPC.lambda;
    m = M2C.m;
    H = CCMPC.H;
    Aineq = CCMPC.Aineq;
    iA = false(2*m, 1);
    options = mpcActiveSetOptions;
    options.MaxIterations = 100;
    options.ConstraintTolerance = 1.0e-5;
end

tic

% Current error tracking
fi = 2 * (Bd') * (-is_ref + Ad * is - Bd * vB);
fi = fi / is_max^2;

% Control action penalization
fv = -2 * vs_ref;
fv = fv / Vc_m_ref^2;

% Complete weighted objective function
f = fi + lambda * fv;

% Control action constraints
ub    = Vc - one_n * vo_ref;
lb    = -one_n * vo_ref;
bineq = [ub; -lb];

% Solve
[vsp, flag, iA, ~] = mpcActiveSetSolver(H, f, Aineq, bineq, zeros(0, m), zeros(0, 1), iA, options);
vs = vsp + one_n * vo_ref;

Tex = toc;
Nac = sum(iA);

is_pred = Ad * is + Bd * (vs - vB);
J_i = sum((is_pred - is_ref).^2) / is_max^2;
J_v = sum((vsp - vs_ref).^2)  / Vc_m_ref^2;
J   = J_i + lambda * J_v;
end

== matlab function Simulate_v2/Predict basic current and voltages ==
  data: VB output; IB output; vxy input; ixy input; ixy_ref input; wy input; RFT parameter; M2C parameter; CEMPC parameter; IB_ref output
function [VB, IB, IB_ref] = pred(vxy, ixy, ixy_ref, wy, RFT, M2C, CEMPC)
%#codegen

% vxy: (p+q) x Np
% ixy: (p+q) x Np
% ixy_ref: (p+q) x Np
% VB: m x Np
% IB: m x Np
% IB_ref: m x Np

persistent p m Np Ts Tab2abc Tabc2ab A pinvA
if isempty(p)
    p       = M2C.p;
    m       = M2C.m;
    Np      = CEMPC.Np;
    Ts      = CEMPC.Ts;
    Tab2abc = RFT.ab2abc;
    Tabc2ab = RFT.abc2ab;
    A      = M2C.A;
    pinvA  = M2C.pinvA;
end

if CEMPC.Np > 1

    %%% Input port
    VX = repmat(vxy(1:p), 1, Np-1);
    IX = repmat(ixy(1:p), 1, Np-1);
    IX_ref = repmat(ixy_ref(1:p), 1, Np-1);

    %%% Output port
    % Rotation matrix
    angles = (1:Np-1) * (wy * Ts);
    cos_vals = cos(angles);
    sin_vals = sin(angles);
    ROTy = reshape([cos_vals; -sin_vals; sin_vals; cos_vals], 2, 2*(Np-1))';

    % Predict
    VY = Tab2abc * reshape(ROTy * Tabc2ab * vxy(p+1:end), 2, Np-1);
    IY = Tab2abc * reshape(ROTy * Tabc2ab * ixy(p+1:end), 2, Np-1);
    IY_ref = Tab2abc * reshape(ROTy * Tabc2ab * ixy_ref(p+1:end), 2, Np-1);

    %%% Predictions formatting
    
    % Concatenate input/output predictions
    VXY = [VX; VY];
    IXY = [IX; IY];
    IXY_ref = [IX_ref; IY_ref];
    
    % Add actual measurement as first predicted step
    VXY = [vxy, VXY];
    IXY = [ixy, IXY];
    IXY_ref = [ixy_ref, IXY_ref];
else
    VXY = vxy;
    IXY = ixy;
    IXY_ref = ixy_ref;
end

% VB = zeros(m, Np);
% IB = zeros(m, Np);
% IB_ref = zeros(m, Np);
VB = zeros(6, 2);
IB = zeros(6, 2);
IB_ref = zeros(6, 2);

VB(:) = A' * VXY;
IB(:) = pinvA * IXY;
IB_ref(:) = pinvA * IXY_ref;

end

== matlab function Simulate_v2/SS cluster voltage reference ==
  data: vs_ref output; iy_ref input; iB_ref input; vB input; wy input; RFT parameter; M2C parameter
function vs_ref = get_vs_ref(iy_ref, iB_ref, vB, wy, RFT, M2C)
%#codegen

persistent rot Tabc2ab Tab2abc pinvA invBs As
if isempty(rot)
    rot = RFT.rot;
    Tabc2ab = RFT.abc2ab;
    Tab2abc = RFT.ab2abc;
    pinvA = M2C.pinvA;
    invBs = M2C.invBs;
    As = M2C.As;
end

dix_ref = [0; 0];
iyab_ref  = Tabc2ab * iy_ref;
diyab_ref = wy * rot * iyab_ref;
diy_ref   = Tab2abc * diyab_ref;
dixy_ref  = [dix_ref; diy_ref];
diB_ref   = pinvA * dixy_ref;
vs_ref = vB + invBs * (diB_ref - As * iB_ref);
end

== matlab function Simulate_v2/MATLAB Function ==
  data: t input; w output; IM parameter
function w = wr_ref(t, IM)

persistent wN wf wi tf ti dw
if isempty(wN)
    wN = IM.wN;
    ti = 0.5;
    tf = 1.5;
    wi = 0;
    wf = wN/10;
    dw = (wf - wi) / (tf - ti);
end

if t < ti
    w = wi;
elseif t < tf
    w = (t - ti) * dw;
else
    w = wf;
end

== matlab function Simulate_v2/Modulation index ==
  data: D output; vs input; Vc input
function D = delta(vs, Vc)
%#codegen

% Modulation index
% D = min(max(vs ./ Vc, 0), 1);
D = (vs ./ Vc);
D = reshape(D, 6, 1);
end
